simulink model "diagrama5"  (R2022a)
settings: Solver=ode45  StartTime=0.0  StopTime=10.0  RelTol=1e-3  EnableMultiTasking=on
libraries: dspobslib x4, dspmathops x2, dspmlti4 x1, commsrccod2 x1, dspsigops x1, dspsrcs4 x1, dspstat3 x1
settings Model: Creator=tcom00  LastModifiedBy=oscar
settings SolverCC: AlgebraicLoopSolver=TrustRegion
settings DataIOCC: LimitDataPoints=on  SaveFormat=Array  SignalLoggingSaveFormat=ModelDataLogs  ReturnWorkspaceOutputs=off  SignalLoggingName=sigsOut
settings OptimizationCC: LifeSpan=inf
settings DebuggingCC: SaveWithParameterizedLinksMsg=none  UnderspecifiedInitializationDetection=Classic  MergeDetectMultiDrivingBlocksExec=none  SignalResolutionControl=TryResolveAllWithWarning  MultiTaskDSMMsg=warning  MultiTaskCondExecSysMsg=none  UnconnectedInputMsg=warning  UnconnectedOutputMsg=warning  UnconnectedLineMsg=warning  AllowSymbolicDim=off  SFUnexpectedBacktrackingDiag=warning  SFNoUnconditionalDefaultTransitionDiag=warning  SFExecutionAtInitializationDiag=none  SFMachineParentedDataDiag=warning  ArithmeticOperatorsInVariantConditions=warning
settings HardwareCC: ProdBitPerPointer=32  ProdBitPerSizeT=32  ProdBitPerPtrDiffT=32  ProdLargestAtomicFloat=None  ProdIntDivRoundTo=Undefined  ProdEndianess=Unspecified  ProdWordSize=32  ProdHWDeviceType=32-bit Generic  TargetUnknown=on
settings ModelReferenceCC: PropagateSignalLabelsOutOfModel=off
settings SFSimCC: SimUseLocalCustomCode=off  CustomCodeUndefinedFunction=UseInterfaceOnly
settings RTWCC: RTWUseLocalCustomCode=off
settings CodeAppCC: StateflowObjectComments=on
settings GRTTargetCC: TargetLangStandard=C89/C90 (ANSI)  CombineOutputUpdateFcns=off  GRTInterface=on
settings ConfigComp: CovMetricSettings=dw  CovSaveCumulativeToWorkspaceVar=on  CovSaveSingleToWorkspaceVar=on  CovExternalEMLEnable=off

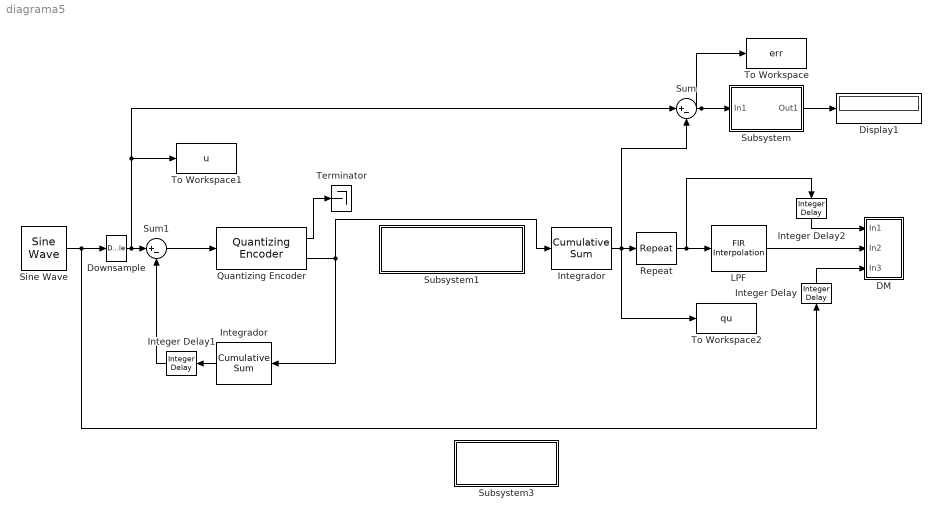
== system diagrama5 ==
  " Integrador " : dspmathops/Cumulative Sum  dim=Channels (running sum)  reset_popup=None  roundingMode=Floor  overflowMode=off  outputDataTypeStr=Inherit: Same as accumulator  outputMin=[]  outputMax=[]  outputLastDataTypeStr=Inherit: Same as accumulator
  DM : Subsystem
      mask Display:
      | plot([0, 1], [1, 1]);
      | plot([0, 0], [1, 0.5]);
      | plot([0, 1], [0.5, 0.5]);
      | plot([1, 1], [1, 0.5]);
      | disp('\n\nMulti\nscope');
  Display1 : Display
  Downsample : DownSample  N=10  RateOptions=Allow multirate processing
  Integer Delay : dspobslib/Integer Delay  delay=50  ic=0  reset_popup=None
      settings: SourceProductBaseCode=DS
  Integer Delay1 : dspobslib/Integer Delay  delay=1  ic=0  reset_popup=None
      settings: SourceProductBaseCode=DS
  Integer Delay2 : dspobslib/Integer Delay  delay=50  ic=0  reset_popup=None
      settings: SourceProductBaseCode=DS
  Integrador : dspmathops/Cumulative Sum  dim=Channels (running sum)  reset_popup=None  roundingMode=Floor  overflowMode=off  outputDataTypeStr=Inherit: Same as accumulator  outputMin=[]  outputMax=[]  outputLastDataTypeStr=Inherit: Same as accumulator
  LPF : dspmlti4/FIR Interpolation  FilterSource=Dialog parameters  PrivateCoeffs=0  h=fir1(101,2.8/100)  L=1  FilterObject=FINTERP  InputProcessing=Columns as channels (frame based)  framing=Allow multirate processing  outputBufInitCond=0  roundingMode=Floor  overflowMode=off  firstCoeffDataTypeStr=Inherit: Same word length as input  firstCoeffMin=[]  firstCoeffMax=[]  firstCoeffLastDataTypeStr=Inherit: Same word length as input  outputDataTypeStr=Inherit: Same as accumulator  outputMin=[]  outputMax=[]  outputLastDataTypeStr=Inherit: Same as accumulator
  Quantizing Encoder : commsrccod2/Quantizing Encoder  partition=[ 0.000000000000: 1.000000000000: 0.000000000000]  codebook=[-0.250000000000, 0.250000000000]  idxDType=double
      settings: SourceProductBaseCode=CM
  Repeat : dspsigops/Repeat  N=4  InputProcessing=Columns as channels (frame based)  RateOptions=Allow multirate processing  ic=0  mode=Unused parameter value
  Sine Wave : dspsrcs4/Sine Wave  Amplitude=1  Frequency=1000  Phase=0  SampleMode=Discrete  OutComplex=Real  CompMethod=Trigonometric fcn  TableSize=Speed  SampleTime=1/200000  SamplesPerFrame=1  ResetState=Restart at time zero  OutputFrames=on  dataType=double  wordLen=16  udDataType=sfix(16)  fracBitsMode=Best precision  numFracBits=14  OutDataTypeStr=double  LastOutDataTypeStr=double
  Subsystem : Subsystem
      mask Display: disp('Running Power');
  Subsystem1 : Subsystem
      mask Display: disp('\nCanal');
  Subsystem3 : Subsystem  mask{delta=0.25}
      mask Callback delta:
      | delta = str2num(get_param(gcb, 'delta'));
      | set_param('diagrama5/Quantizing Encoder', 'Codebook', ['[', sprintf('%15.12f',-delta), ',', sprintf('%15.12f',delta), ']']);
      mask Display: disp('Parametros del\nsistema');
  Sum : Sum  Inputs=|+-  SaturateOnIntegerOverflow=on
  Sum1 : Sum  Inputs=|+-  SaturateOnIntegerOverflow=on
  Terminator : Terminator
  To Workspace : ToWorkspace  VariableName=err  SampleTime=-1
      settings: Save2DSignal=2-D array (concatenate along first dimension)
  To Workspace1 : ToWorkspace  VariableName=u  SampleTime=-1
      settings: Save2DSignal=2-D array (concatenate along first dimension)
  To Workspace2 : ToWorkspace  VariableName=qu  SampleTime=-1
      settings: Save2DSignal=2-D array (concatenate along first dimension)
  wires:
  Sine Wave/1 -> Downsample/1, Integer Delay/1
  Downsample/1 -> Sum/1, To Workspace1/1, Sum1/1
  Quantizing Encoder/2 -> Integrador/1, " Integrador "/1
  Integrador/1 -> Integer Delay1/1
  Integer Delay1/1 -> Sum1/2
  Repeat/1 -> LPF/1, Integer Delay2/1
  Sum/1 -> Subsystem/1(In1), To Workspace/1
  Integer Delay/1 -> DM/3(In3)
  LPF/1 -> DM/2(In2)
  Integer Delay2/1 -> DM/1(In1)
  Sum1/1 -> Quantizing Encoder/1
  Quantizing Encoder/1 -> Terminator/1
  " Integrador "/1 -> Sum/2, To Workspace2/1, Repeat/1
  Subsystem/1(Out1) -> Display1/1

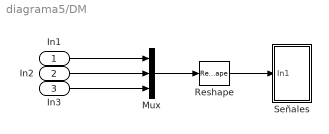
== system diagrama5/DM ==
  In1 : Inport
  In2 : Inport  Port=2
  In3 : Inport  Port=3
  Mux : Mux  Inputs=3
  Reshape : Reshape  OutputDimensionality=Row vector (2-D)
  Señales : Subsystem
      mask Display:
      | plot([0, 1], [1, 1]);
      | plot([0, 0], [1, 0.5]);
      | plot([0, 1], [0.5, 0.5]);
      | plot([1, 1], [1, 0.5]);
      | disp('\n\nFrame\nscope');
  wires:
  Mux/1 -> Reshape/1
  Reshape/1 -> Señales/1(In1)
  In1/1 -> Mux/1
  In2/1 -> Mux/2
  In3/1 -> Mux/3

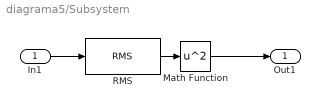
== system diagrama5/Subsystem ==
  In1 : Inport
  Math Function : Math  Operator=square  SignedPower=on
  RMS : dspstat3/RMS  run=on  directionMode=Each row  dimension=1  reset_popup=None
  Out1 : Outport  VectorParamsAs1DForOutWhenUnconnected=off
  wires:
  RMS/1 -> Math Function/1
  In1/1 -> RMS/1
  Math Function/1 -> Out1/1

== system diagrama5/Subsystem1 ==

== system diagrama5/Subsystem3 ==

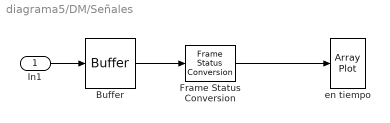
== system diagrama5/DM/Señales ==
  In1 : Inport
  Buffer : Buffer  N=500
  Frame Status Conversion : dspobslib/Frame Status Conversion  growRefPort=off  outframe=Frame-based
      settings: SourceProductBaseCode=DS
  en tiempo : ArrayPlot  WindowPosition=[566.000000,483.000000,658.000000,431.000000,]  ScopeFrameLocation=window  PlotType=Line  XLabel=Tiempo (s)  YLabel=Amplitud  YLimits=[-1.5313,1.2813]  ShowLegend=on
  wires:
  Buffer/1 -> Frame Status Conversion/1
  Frame Status Conversion/1 -> en tiempo/1
  In1/1 -> Buffer/1
